simulink model "buck_dev_perturb"  (R2024a)
settings: Solver=ode23t  StartTime=0.0  StopTime=0.25  MaxStep=5e-7  RelTol=1e-3
values from neighbouring files (symbols this model uses):
  Cf = 1/(Lf*(0.1*2*pi*fs)^2)    (= 2.41240913434e-06)    [buck_control_design.m]    (also in buck_control_init.m = 9.64963653737e-06; buck_conv_code.m = 9.64963653737e-06; buck_conv_code_1.m = 1 / (Lf * (0.05 * 2 * pi * fs)^2); buck_impedance_scan_init.m = 9.64963653737e-06)
  D0 = Uout0/Vdc0    (= 0.571428571429)    [buck_conv_code.m]    (also in buck_conv_code_1.m = Uout0 / Vdc0; buck_impedance_scan_init.m)
  fsamp = 24e3    (= 24000)    [buck_control_design.m]    (also in buck_control_init.m = 48000; buck_conv_code.m = 48000; buck_conv_code_1.m = 48000; buck_impedance_scan_init.m = 48000)
  Imax = 2*Iload0    (= 40)    [buck_control_init.m]    (also in buck_conv_code.m; buck_conv_code_1.m = 2 * Iload0; buck_impedance_scan_init.m)
  kpi = wBWi*Lf    (= 27.4889357189)    [buck_control_design.m]    (also in buck_control_init.m = 9.62112750162; buck_conv_code.m = 9.62112750162; buck_conv_code_1.m = wBWi * Lf; buck_impedance_scan_init.m = 9.62112750162)
  kpu = wBWu*Cf    (= 0.00363782727067)    [buck_control_design.m]    (also in buck_control_init.m = 0.0203718327158; buck_conv_code.m = 0.0203718327158; buck_conv_code_1.m = wBWu * Cf; buck_impedance_scan_init.m = 0.0203718327158)
  kuff = 1    [buck_control_design.m]    (also in buck_control_init.m; buck_conv_code.m; buck_conv_code_1.m; buck_impedance_scan_init.m)
  Lf = 1/fs*1/(0.4*Iload0)*(1-0.5)*Vdc0    (= 0.00182291666667)    [buck_control_design.m]    (also in buck_control_init.m = 0.000455729166667; buck_conv_code.m = 0.000455729166667; buck_conv_code_1.m = 0.5 * 1 / (fs) * 1 / (0.2 * Iload0) * (1 - 0.5) * Vdc0; buck_impedance_scan_init.m = 0.000455729166667)
  Tsamp = 1/fsamp    (= 2.08333333333e-05)    [buck_control_init.m]    (also in buck_conv_code.m; buck_conv_code_1.m; buck_impedance_scan_init.m)
  uRef0 = Uout0    (= 200)    [buck_control_design.m]    (also in buck_control_init.m; buck_conv_code.m; buck_conv_code_1.m = Uout0; buck_impedance_scan_init.m)
  Vdc0 = 350    [buck_control_design.m]    (also in buck_control_init.m; buck_conv_code.m; buck_conv_code_1.m; buck_impedance_scan_init.m)
libraries: simulink x4, spsSeriesRLCBranchLib x3, spsCurrentMeasurementLib x2, spsDCVoltageSourceLib x1, spsDiodeLib x1, spsIGBTDiodeLib x1, spsVoltageMeasurementLib x1, sps_lib x1
settings Model: Creator=CHMASCH32  LastModifiedBy=nawaz
settings OptimizationCC: ReuseModelBlockBuffer=off
settings RTWCC: GPUComputeCapability=3.5

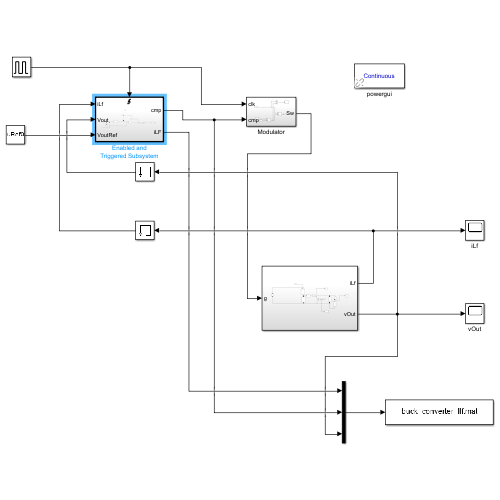
[thumbnail: Simulink's stored preview of the top-level diagram]
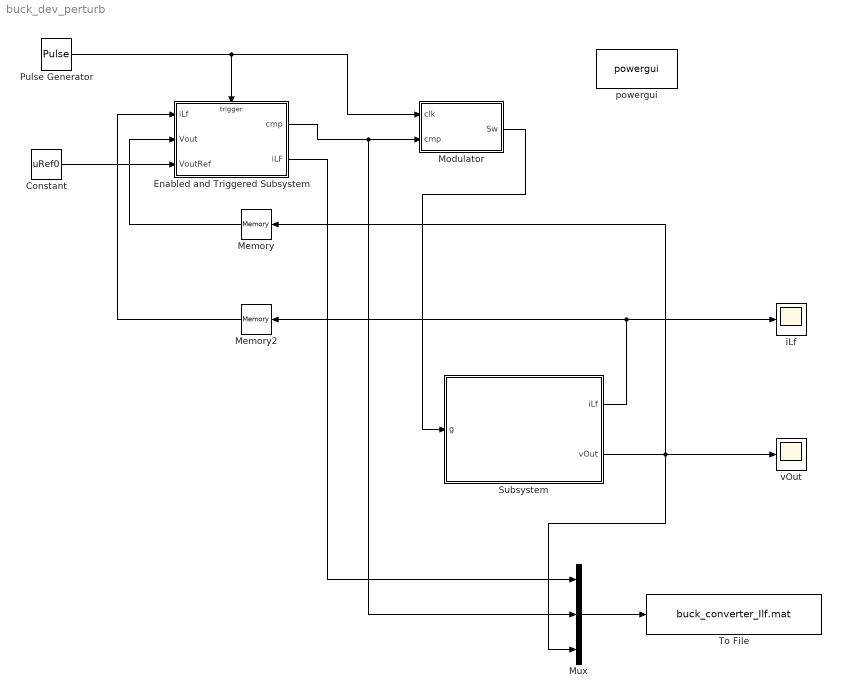
== system buck_dev_perturb ==
  Constant : Constant  Value=uRef0
  Enabled and Triggered Subsystem : Subsystem  TreatAsAtomicUnit=on
  Memory : Memory
  Memory2 : Memory
  Modulator : Subsystem
  Mux : Mux  Inputs=3
  Pulse Generator : DiscretePulseGenerator  PulseType=Time based  Period=Tsamp  PulseWidth=50
  Subsystem : Subsystem
  To File : ToFile  Filename=buck_converter_Ilf.mat  MatrixName=Ilf  SaveFormat=Timeseries
  iLf : Scope
  powergui : sps_lib/powergui  Priority=1  SimulationMode=Continuous  SampleTime=50e-6  frequency=60  Iterations=50  frequencyindice=0  Pbase=100e6  ErrMax=1e-4  UnitsV=kV  UnitsW=MW  buscounter=0  FunctionMessages=off  echomessages=off  EnableUseOfTLC=off  CurrentSourceSwitches=off  DisableSnubberDevices=off  DisableRonSwitches=off  DisableVfSwitches=off  DisplayEquations=off  AutomaticDiscreteSolvers=off  SolverType=Tustin/Backward Euler (TBE)  Interpol=off  ExternalGateDelay=off  methode=off  Ts=100  x0status=blocks  SPID=on  SwTol=0  HookPort=off  NonlinearTolerance=1e-4  nMaxIteration=100  ContinueOnMaxIteration=off  RestoreLinks=warning  ResistiveCurrentMeasurement=off  Frange=[0:2:500]  Ylog=off  Xlog=on  ShowGrid=off  save=off  variable=ZData  structure=0  ZoomFFT=off  StartTime=0.0  cycles=1  DisplayStyle=1  fundamental=60  FreqAxis=off  MaxFrequency=1000  frequencyindicesteady=1  RmsSteady=1  display=off
  vOut : Scope
  wires:
  Pulse Generator/1 -> Enabled and Triggered Subsystem/Trigger, Modulator/1(clk)
  Enabled and Triggered Subsystem/1(cmp) -> Mux/2, Modulator/2(cmp)
  Modulator/1(Sw) -> Subsystem/1(g)
  Subsystem/1(iLf) -> iLf/1, Memory2/1
  Constant/1 -> Enabled and Triggered Subsystem/3(VoutRef)
  Memory/1 -> Enabled and Triggered Subsystem/2(Vout)
  Memory2/1 -> Enabled and Triggered Subsystem/1(iLf)
  Subsystem/2(vOut) -> Mux/3, Memory/1, vOut/1
  Mux/1 -> To File/1
  Enabled and Triggered Subsystem/2(iLF) -> Mux/1

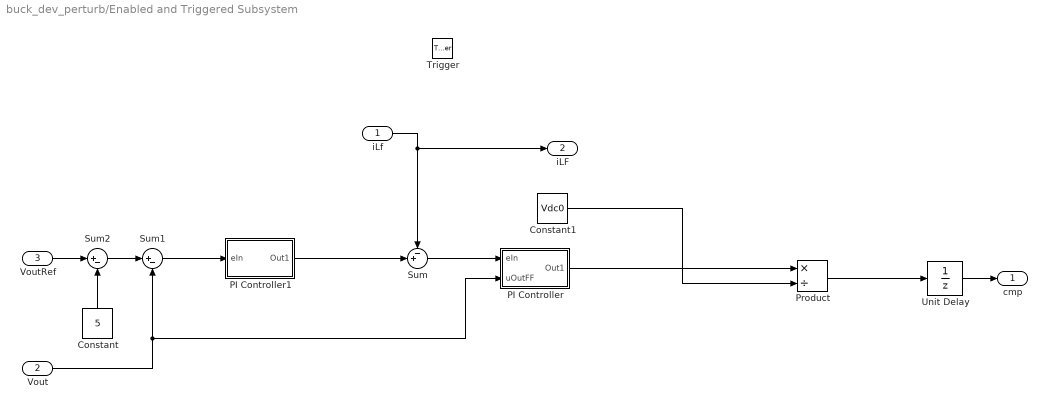
== system buck_dev_perturb/Enabled and Triggered Subsystem ==
  iLf : Inport
  Vout : Inport  Port=2
  VoutRef : Inport  Port=3
  Trigger : TriggerPort  VariantControl=(inherit)
  Constant : Constant  Value=5
  Constant1 : Constant  Value=Vdc0
  PI Controller : Subsystem
  PI Controller1 : Subsystem
  Product : Product  Inputs=*/
  Sum : Sum  Inputs=-+|
  Sum1 : Sum  Inputs=|+-
  Sum2 : Sum  Inputs=|+-
  Unit Delay : UnitDelay  InitialCondition=D0  SampleTime=-1  HasFrameUpgradeWarning=on
  cmp : Outport
  iLF : Outport  Port=2
  wires:
  Unit Delay/1 -> cmp/1
  Sum/1 -> PI Controller/1(eIn)
  iLf/1 -> Sum/1, iLF/1
  Vout/1 -> Sum1/2, PI Controller/2(uOutFF)
  Sum1/1 -> PI Controller1/1(eIn)
  PI Controller/1(Out1) -> Product/1
  Product/1 -> Unit Delay/1
  Constant1/1 -> Product/2
  PI Controller1/1(Out1) -> Sum/2
  Sum2/1 -> Sum1/1
  VoutRef/1 -> Sum2/1
  Constant/1 -> Sum2/2

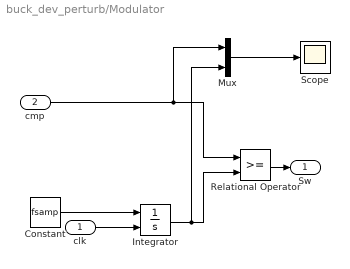
== system buck_dev_perturb/Modulator ==
  clk : Inport
  cmp : Inport  Port=2
  Constant : Constant  Value=fsamp
  Integrator : Integrator  ExternalReset=rising
  Mux : Mux  Inputs=2
  Relational Operator : RelationalOperator  OutDataTypeStr=boolean  RndMeth=Simplest  InputSameDT=off
  Scope : Scope
  Sw : Outport
  wires:
  Constant/1 -> Integrator/1
  Integrator/1 -> Mux/2, Relational Operator/2
  Relational Operator/1 -> Sw/1
  clk/1 -> Integrator/2
  cmp/1 -> Mux/1, Relational Operator/1
  Mux/1 -> Scope/1

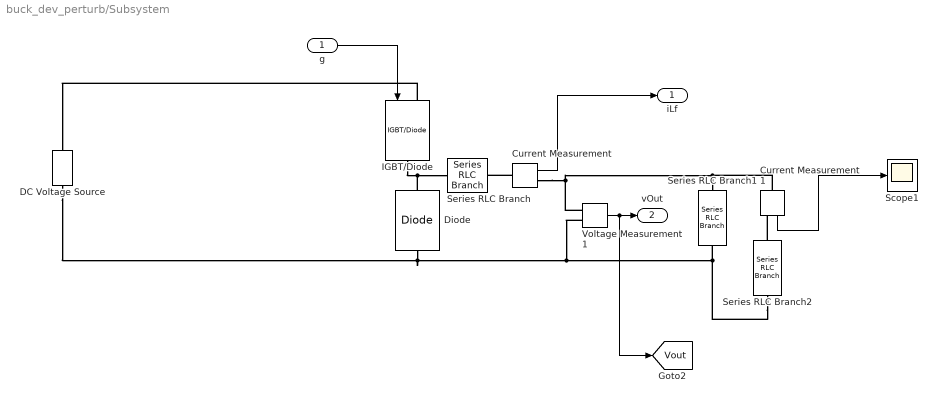
== system buck_dev_perturb/Subsystem ==
  g : Inport
  Current Measurement : spsCurrentMeasurementLib/Current Measurement  PhasorSimulation=off  OutputType=Complex  PSBequivalent=0
  Current Measurement1 : spsCurrentMeasurementLib/Current Measurement  PhasorSimulation=off  OutputType=Complex  PSBequivalent=0
  DC Voltage Source : spsDCVoltageSourceLib/DC Voltage Source  Amplitude=Vdc0  Measurements=None
  Diode : spsDiodeLib/Diode  Ron=0.0001  Lon=0  Vf=0  IC=0  UseSnubber=0  Rs=1e5  Cs=inf  Measurements=off
  IGBT/Diode : spsIGBTDiodeLib/IGBT//Diode  Ron=1e-4  Rs=1e5  Cs=inf  Measurements=off
  Scope1 : Scope
  Series RLC Branch : spsSeriesRLCBranchLib/Series RLC Branch  LConnTagsString=__new0  RConnTagsString=__new0  BranchType=L  Resistance=1  Inductance=Lf  SetiL0=on  InitialCurrent=iLf0  Capacitance=1e-6  Setx0=off  InitialVoltage=0  Measurements=None
  Series RLC Branch1 : spsSeriesRLCBranchLib/Series RLC Branch  LConnTagsString=__new0  RConnTagsString=__new0  BranchType=C  Resistance=1  Inductance=1e-3  SetiL0=off  InitialCurrent=0  Capacitance=Cf  Setx0=on  InitialVoltage=Uout0  Measurements=None
  Series RLC Branch2 : spsSeriesRLCBranchLib/Series RLC Branch  LConnTagsString=__new0  RConnTagsString=__new0  BranchType=R  Resistance=10  Inductance=1e-3  SetiL0=off  InitialCurrent=0  Capacitance=Cf  Setx0=on  InitialVoltage=Uout0  Measurements=None
  Voltage Measurement1 : spsVoltageMeasurementLib/Voltage Measurement  PhasorSimulation=off  OutputType=Complex  PSBequivalent=0
  iLf : Outport
  vOut : Outport  Port=2
  tag scope: Vout=global
  wires:
  Voltage Measurement1/1 -> [Vout], vOut/1
  g/1 -> IGBT/Diode/1
  Current Measurement1/1 -> Scope1/1
  Current Measurement/1 -> iLf/1
  connections:
  Voltage Measurement1/LConn1 -- Current Measurement/RConn1 -- Current Measurement1/LConn1 -- Series RLC Branch1/LConn1
  IGBT/Diode/RConn1 -- Series RLC Branch/LConn1 -- Diode/RConn1
  DC Voltage Source/LConn1 -- Voltage Measurement1/LConn2 -- Series RLC Branch2/RConn1 -- Series RLC Branch1/RConn1 -- Diode/LConn1
  Current Measurement/LConn1 -- Series RLC Branch/RConn1
  IGBT/Diode/LConn1 -- DC Voltage Source/RConn1
  Series RLC Branch2/LConn1 -- Current Measurement1/RConn1

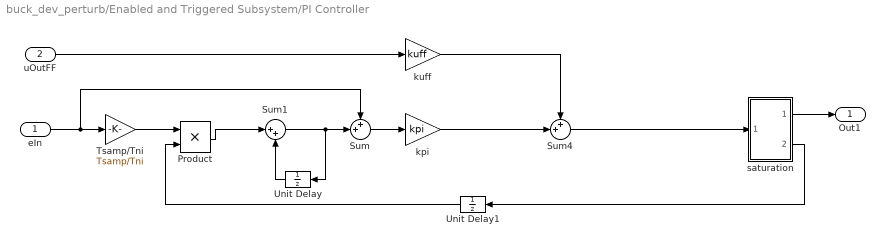
== system buck_dev_perturb/Enabled and Triggered Subsystem/PI Controller ==
  eIn : Inport
  uOutFF : Inport  Port=2
  Product : Product  OutDataTypeStr=double  RndMeth=Zero
  Sum : Sum  Inputs=++|
  Sum1 : Sum  Inputs=|++
  Sum4 : Sum  Inputs=++|
  Tsamp/Tni : Gain  Gain=Tsamp/Tni  OutDataTypeStr=double
  Unit Delay : UnitDelay  SampleTime=-1  HasFrameUpgradeWarning=on
  Unit Delay1 : UnitDelay  SampleTime=-1  HasFrameUpgradeWarning=on
  kpi : Gain  Gain=kpi
  kuff : Gain  Gain=kuff
  saturation : Subsystem
  Out1 : Outport  VectorParamsAs1DForOutWhenUnconnected=off
  wires:
  Sum/1 -> kpi/1
  Tsamp/Tni/1 -> Product/1
  saturation/1(sig_sat) -> Out1/1
  Sum4/1 -> saturation/1(sig_in)
  uOutFF/1 -> kuff/1
  Sum1/1 -> Sum/2, Unit Delay/1
  Unit Delay/1 -> Sum1/2
  Product/1 -> Sum1/1
  kuff/1 -> Sum4/1
  kpi/1 -> Sum4/2
  saturation/2(!sat) -> Unit Delay1/1
  Unit Delay1/1 -> Product/2
  eIn/1 -> Tsamp/Tni/1, Sum/1

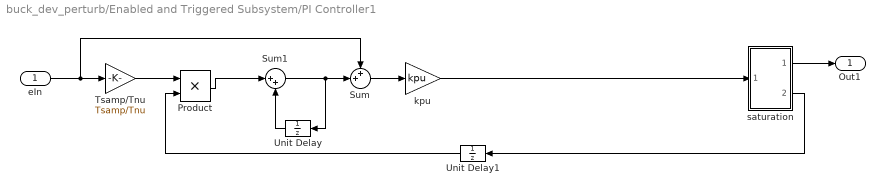
== system buck_dev_perturb/Enabled and Triggered Subsystem/PI Controller1 ==
  eIn : Inport
  Product : Product  OutDataTypeStr=double  RndMeth=Zero
  Sum : Sum  Inputs=++|
  Sum1 : Sum  Inputs=|++
  Tsamp/Tnu : Gain  Gain=Tsamp/Tnu  OutDataTypeStr=double
  Unit Delay : UnitDelay  SampleTime=-1  HasFrameUpgradeWarning=on
  Unit Delay1 : UnitDelay  SampleTime=-1  HasFrameUpgradeWarning=on
  kpu : Gain  Gain=kpu
  saturation : Subsystem
  Out1 : Outport  VectorParamsAs1DForOutWhenUnconnected=off
  wires:
  eIn/1 -> Sum/1, Tsamp/Tnu/1
  Unit Delay1/1 -> Product/2
  saturation/2(!sat) -> Unit Delay1/1
  Product/1 -> Sum1/1
  Unit Delay/1 -> Sum1/2
  Sum1/1 -> Unit Delay/1, Sum/2
  saturation/1(sig_sat) -> Out1/1
  Tsamp/Tnu/1 -> Product/1
  Sum/1 -> kpu/1
  kpu/1 -> saturation/1(sig_in)

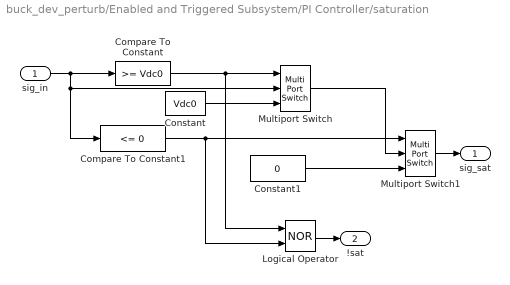
== system buck_dev_perturb/Enabled and Triggered Subsystem/PI Controller/saturation ==
  sig_in : Inport
  Compare To Constant : simulink/Logic and Bit Operations/Compare To Constant  relop=>=  const=Vdc0  OutDataTypeStr=boolean  ZeroCross=off
  Compare To Constant1 : simulink/Logic and Bit Operations/Compare To Constant  relop=<=  const=0  OutDataTypeStr=boolean  ZeroCross=off
  Constant : Constant  Value=Vdc0
  Constant1 : Constant  Value=0
  Logical Operator : Logic  Operator=NOR  AllPortsSameDT=off  OutDataTypeStr=boolean
  Multiport Switch : MultiPortSwitch  DataPortOrder=Zero-based contiguous  Inputs=2  zeroidx=on  SaturateOnIntegerOverflow=off  InputSameDT=off
  Multiport Switch1 : MultiPortSwitch  DataPortOrder=Zero-based contiguous  Inputs=2  zeroidx=on  SaturateOnIntegerOverflow=off  InputSameDT=off
  sig_sat : Outport  VectorParamsAs1DForOutWhenUnconnected=off
  !sat : Outport  Port=2  VectorParamsAs1DForOutWhenUnconnected=off
  wires:
  Compare To Constant/1 -> Multiport Switch/1, Logical Operator/1
  sig_in/1 -> Compare To Constant/1, Multiport Switch/2, Compare To Constant1/1
  Compare To Constant1/1 -> Multiport Switch1/1, Logical Operator/2
  Multiport Switch/1 -> Multiport Switch1/2
  Constant1/1 -> Multiport Switch1/3
  Constant/1 -> Multiport Switch/3
  Multiport Switch1/1 -> sig_sat/1
  Logical Operator/1 -> !sat/1

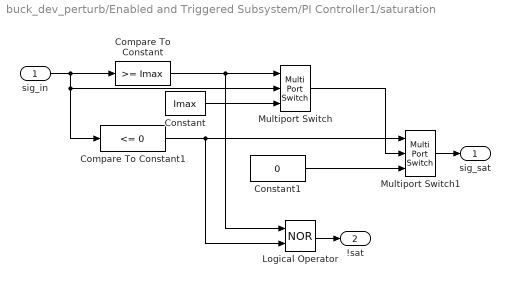
== system buck_dev_perturb/Enabled and Triggered Subsystem/PI Controller1/saturation ==
  sig_in : Inport
  Compare To Constant : simulink/Logic and Bit Operations/Compare To Constant  relop=>=  const=Imax  OutDataTypeStr=boolean  ZeroCross=off
  Compare To Constant1 : simulink/Logic and Bit Operations/Compare To Constant  relop=<=  const=0  OutDataTypeStr=boolean  ZeroCross=off
  Constant : Constant  Value=Imax
  Constant1 : Constant  Value=0
  Logical Operator : Logic  Operator=NOR  AllPortsSameDT=off  OutDataTypeStr=boolean
  Multiport Switch : MultiPortSwitch  DataPortOrder=Zero-based contiguous  Inputs=2  zeroidx=on  SaturateOnIntegerOverflow=off  InputSameDT=off
  Multiport Switch1 : MultiPortSwitch  DataPortOrder=Zero-based contiguous  Inputs=2  zeroidx=on  SaturateOnIntegerOverflow=off  InputSameDT=off
  sig_sat : Outport  VectorParamsAs1DForOutWhenUnconnected=off
  !sat : Outport  Port=2  VectorParamsAs1DForOutWhenUnconnected=off
  wires:
  Logical Operator/1 -> !sat/1
  Multiport Switch1/1 -> sig_sat/1
  Constant/1 -> Multiport Switch/3
  Constant1/1 -> Multiport Switch1/3
  Multiport Switch/1 -> Multiport Switch1/2
  Compare To Constant1/1 -> Logical Operator/2, Multiport Switch1/1
  sig_in/1 -> Compare To Constant1/1, Multiport Switch/2, Compare To Constant/1
  Compare To Constant/1 -> Logical Operator/1, Multiport Switch/1
